simulink model "ex1_1"  (R2021a)
settings: Solver=VariableStepAuto  StartTime=0.0  StopTime=simTime  RelTol=1e-3
values from neighbouring files (symbols this model uses):
  alpha = deg2rad(10)    [ex1_1_variables.m]
  g = 9.81    [ex1_1_variables.m]
  Ka1 = 1250/3    (= 416.666666667)    [ex1_1_variables.m]
  Kmv = 0.18    [ex1_1_variables.m]
  Kp = 20    [ex1_1_variables.m]
  m = 1500    [ex1_1_variables.m]
  tSlope = 15    [ex1_1_variables.m]
  vc = vc/3.6/Kp    (= 1.11111111111)    [ex1_1_variables.m]
settings Model: Creator=ocean  LastModifiedBy=ocean

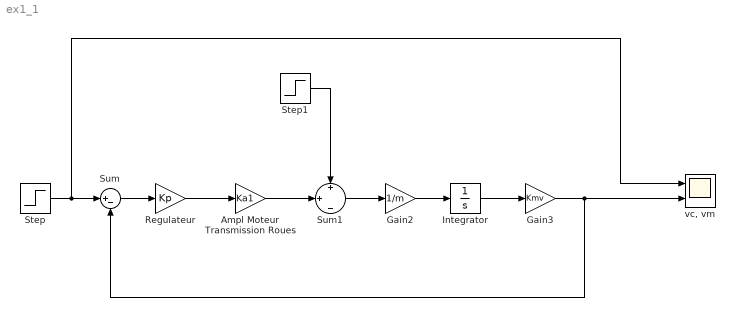
== system ex1_1 ==
  "Ampl Moteur Transmission Roues " : Gain  Gain=Ka1
  Gain2 : Gain  Gain=1/m
  Gain3 : Gain  Gain=Kmv
  Integrator : Integrator
  Regulateur : Gain  Gain=Kp
  Step : Step  After=vc  SampleTime=0
  Step1 : Step  Time=tSlope  After=-m*g*sin(alpha)  SampleTime=0
  Sum : Sum  Inputs=|+-
  Sum1 : Sum  Inputs=+|+|-
  "vc, vm" : Scope  NumInputPorts=2
  wires:
  Regulateur/1 -> "Ampl Moteur Transmission Roues "/1
  Sum/1 -> Regulateur/1
  "Ampl Moteur Transmission Roues "/1 -> Sum1/2
  Sum1/1 -> Gain2/1
  Gain2/1 -> Integrator/1
  Integrator/1 -> Gain3/1
  Gain3/1 -> Sum/2, "vc, vm"/2
  Step/1 -> "vc, vm"/1, Sum/1
  Step1/1 -> Sum1/1
